simulink model "Problem4"  (R2020b)
settings: Solver=VariableStepAuto  StartTime=0.0  StopTime=10.0  RelTol=1e-3
settings Model: Creator=Shirish  LastModifiedBy=Shirish

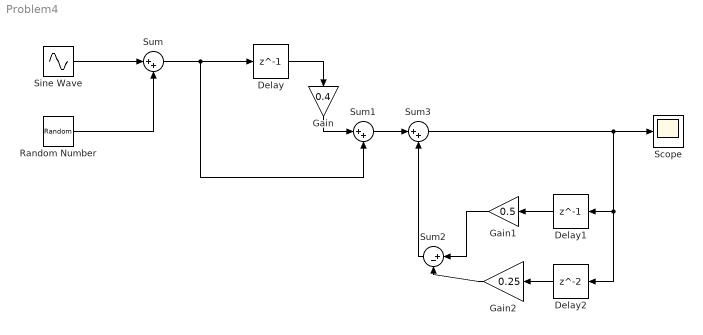
== system Problem4 ==
  Delay : Delay  DelayLength=1
  Delay1 : Delay  DelayLength=1
  Delay2 : Delay
  Gain : Gain  Gain=0.4
  Gain1 : Gain  Gain=0.5
  Gain2 : Gain  Gain=0.25
  Random Number : RandomNumber  SampleTime=0.1
  Scope : Scope
  Sine Wave : Sin  SampleTime=0
  Sum : Sum  Inputs=|++
  Sum1 : Sum  Inputs=|++
  Sum2 : Sum  Inputs=|+-
  Sum3 : Sum  Inputs=|++
  wires:
  Sine Wave/1 -> Sum/1
  Random Number/1 -> Sum/2
  Sum/1 -> Sum1/2, Delay/1
  Delay/1 -> Gain/1
  Gain/1 -> Sum1/1
  Delay2/1 -> Gain2/1
  Delay1/1 -> Gain1/1
  Gain1/1 -> Sum2/1
  Gain2/1 -> Sum2/2
  Sum1/1 -> Sum3/1
  Sum2/1 -> Sum3/2
  Sum3/1 -> Delay2/1, Delay1/1, Scope/1
